simulink model "ilc_drone"  (Simulink 9.1)
settings: Solver=ode45  StartTime=0.0  StopTime=900  RelTol=1e-3  EnableMultiTasking=on
libraries: simulink_need_slupdate x1
settings Model: Creator=aeagr  LastModifiedBy=aeagr
settings DataIOCC: LimitDataPoints=on  SignalLoggingSaveFormat=ModelDataLogs
settings OptimizationCC: ExpressionDepthLimit=2147483647
settings DebuggingCC: SolverPrmCheckMsg=warning  FcnCallInpInsideContextMsg=warning  StateNameClashWarn=warning
settings GRTTargetCC: GeneratePreprocessorConditionals=Disable all  CombineOutputUpdateFcns=on  GRTInterface=off

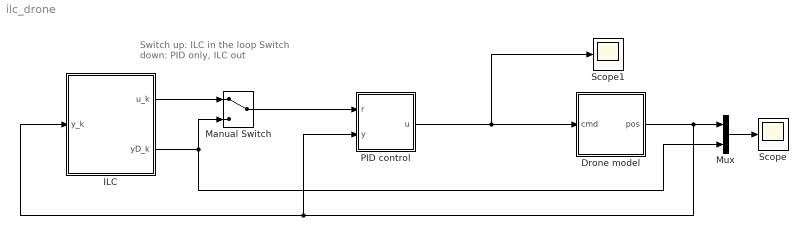
== system ilc_drone ==
  note: Switch up: ILC in the loop
      | Switch down: PID only, ILC out
  Drone model : Subsystem
  ILC : Subsystem  Description=Iterative Learning Control  TreatAsAtomicUnit=on  SystemSampleTime=dt  mask{Yseq=kron([1 0 -1 0],sin((1:30)*2*pi/60).^3), dt=1, gamma=0.3}
      mask prompts: Yseq "Target output sequence"; dt "Time step"; gamma "Learning rate"
  Manual Switch : ManualSwitch
  Mux : Mux  Inputs=2
  PID control : Subsystem
  Scope : Scope
  Scope1 : Scope
  wires:
  Mux/1 -> Scope/1
  ILC/2(yD_k) -> Manual Switch/2, Mux/2
  ILC/1(u_k) -> Manual Switch/1
  PID control/1(u) -> Scope1/1, Drone model/1(cmd)
  Manual Switch/1 -> PID control/1(r)
  Drone model/1(pos) -> PID control/2(y), ILC/1(y_k), Mux/1

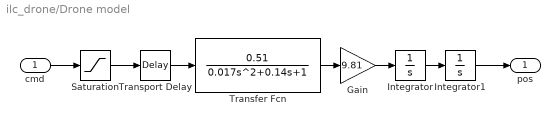
== system ilc_drone/Drone model ==
  cmd : Inport
  Gain : Gain  Gain=9.81
  Integrator : Integrator
  Integrator1 : Integrator
  Saturation : Saturate  UpperLimit=0.37  LowerLimit=-0.37
  Transfer Fcn : TransferFcn  Numerator=0.51  Denominator=[0.017 0.14 1]
  Transport Delay : TransportDelay  DelayTime=0.75
  pos : Outport
  wires:
  Integrator/1 -> Integrator1/1
  Transport Delay/1 -> Transfer Fcn/1
  cmd/1 -> Saturation/1
  Gain/1 -> Integrator/1
  Transfer Fcn/1 -> Gain/1
  Saturation/1 -> Transport Delay/1
  Integrator1/1 -> pos/1

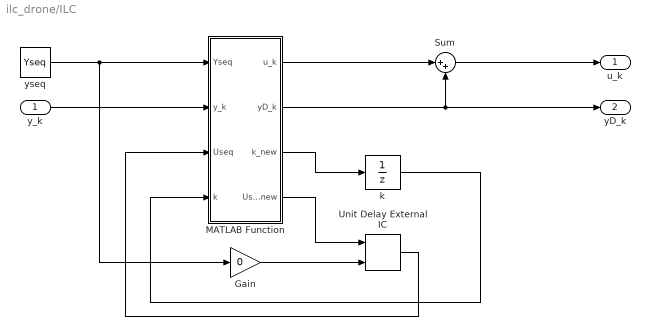
== system ilc_drone/ILC ==
  y_k : Inport
  Gain : Gain  Gain=0
  MATLAB Function : MATLAB Function  TreatAsAtomicUnit=on
  Sum : Sum  Inputs=|++
  Unit Delay External IC : simulink_need_slupdate/Unit Delay External IC  tsamp=-1
      settings: SourceProductName=Simulink  SourceProductBaseCode=SL
  k : UnitDelay  InitialCondition=1  SampleTime=-1
  yseq : Constant  Value=Yseq
  u_k : Outport
  yD_k : Outport  Port=2
  wires:
  MATLAB Function/3(k_new) -> k/1
  MATLAB Function/4(Useq_new) -> Unit Delay External IC/1
  Unit Delay External IC/1 -> MATLAB Function/3(Useq)
  y_k/1 -> MATLAB Function/2(y_k)
  yseq/1 -> MATLAB Function/1(Yseq), Gain/1
  k/1 -> MATLAB Function/4(k)
  MATLAB Function/2(yD_k) -> Sum/2, yD_k/1
  Sum/1 -> u_k/1
  MATLAB Function/1(u_k) -> Sum/1
  Gain/1 -> Unit Delay External IC/2

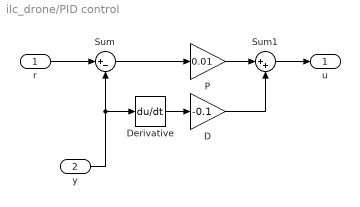
== system ilc_drone/PID control ==
  r : Inport
  y : Inport  Port=2
  D : Gain  Gain=-0.1
  Derivative : Derivative  CoefficientInTFapproximation=0.001
  P : Gain  Gain=0.01
  Sum : Sum  Inputs=|+-
  Sum1 : Sum  Inputs=|++
  u : Outport
  wires:
  Sum/1 -> P/1
  Derivative/1 -> D/1
  P/1 -> Sum1/1
  y/1 -> Sum/2, Derivative/1
  r/1 -> Sum/1
  Sum1/1 -> u/1
  D/1 -> Sum1/2

== matlab function ILC/MATLAB Function ==
  data: u_k output double; Yseq input double; yD_k output double; y_k input double; Useq input double; k input double; k_new output double; Useq_new output double; gamma parameter double
function [u_k,yD_k,k_new,Useq_new] = fcn(Yseq,y_k,Useq,k,gamma)
%#codegen

% number of elements in sequence
Nseq = numel(Yseq);

% counter
k_new = k+1;
% reset if we've been round the sequence
if k_new>Nseq,
    k_new=1;
end

% extract current demand signal
yD_k = Yseq(k);

% and the current control
u_k = Useq(k);

% form the error
e_k = yD_k - y_k;

% copy the control sequence over
Useq_new = Useq;

% which entry to update
k_learn = k-1;
if k_learn<1,
    k_learn=Nseq;
end

% do the learning update
Useq_new(k_learn) = Useq_new(k_learn) + gamma*e_k;
